simulink model "Simulink_Simulation"  (R2020a)
settings: Solver=ode23tb  StartTime=0.0  StopTime=10.0  RelTol=1e-3  EnableMultiTasking=on
undefined symbols (not defined in the file or in its folder): sigbuilder_block
libraries: powerlib x8
settings Model: Creator=LENOVO  LastModifiedBy=x64
settings DataIOCC: LimitDataPoints=on  SaveFormat=Array  ReturnWorkspaceOutputs=off
settings OptimizationCC: LifeSpan=inf
settings DebuggingCC: SolverPrmCheckMsg=warning  SFUnexpectedBacktrackingDiag=warning  SFNoUnconditionalDefaultTransitionDiag=warning  SFExecutionAtInitializationDiag=none  ArithmeticOperatorsInVariantConditions=warning
settings HardwareCC: ProdBitPerPointer=32  ProdBitPerSizeT=32  ProdBitPerPtrDiffT=32  ProdLargestAtomicFloat=None  ProdIntDivRoundTo=Undefined  ProdEndianess=Unspecified  ProdWordSize=32  ProdHWDeviceType=32-bit Generic
settings ModelReferenceCC: PropagateSignalLabelsOutOfModel=off
settings SFSimCC: SimUseLocalCustomCode=off  CustomCodeUndefinedFunction=UseInterfaceOnly
settings RTWCC: RTWUseLocalCustomCode=off
settings CodeAppCC: StateflowObjectComments=on
settings GRTTargetCC: TargetLangStandard=C89/C90 (ANSI)
settings ConfigComp: CovMetricSettings=dw  CovHtmlReporting=on  CovSaveCumulativeToWorkspaceVar=on  CovSaveSingleToWorkspaceVar=on  CovExternalEMLEnable=off  CovSFcnEnable=off
settings SimscapeCC: SimscapeNormalizeSystem=off

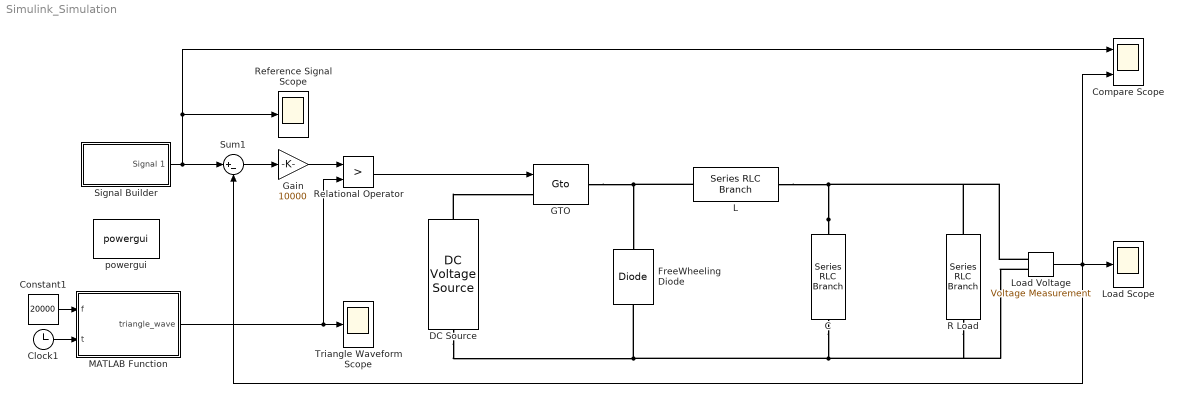
== system Simulink_Simulation ==
  "C " : powerlib/Elements/Series RLC Branch  LConnTagsString=__new0  RConnTagsString=__new0  BranchType=C  Resistance=1  Inductance=1e-3  SetiL0=off  InitialCurrent=0  Capacitance=(1e-6)*470  Setx0=off  InitialVoltage=0  Measurements=None
  Clock1 : Clock
  Compare Scope : Scope  NumInputPorts=2
  Constant1 : Constant  Value=20000
  "DC Source " : powerlib/Electrical Sources/DC Voltage Source  Amplitude=15  Measurements=None
  FreeWheeling Diode : powerlib/Power Electronics/Diode  Ron=0.01  Lon=1e-4  Vf=0.8  IC=0  UseSnubber=off  Rs=10000  Cs=1e-4  Measurements=off
  GTO : powerlib/Power Electronics/Gto  Ron=0.01  Lon=0.001  Vf=0.8  Tf=10e-6  Tt=20e-6  IC=0  Rs=10000  Cs=1e-5  Measurements=off
      settings: SourceProductBaseCode=PS
  Gain : Gain  Gain=10000
  L : powerlib/Elements/Series RLC Branch  LConnTagsString=__new0  RConnTagsString=__new0  BranchType=L  Resistance=1  Inductance=1e-4  SetiL0=off  InitialCurrent=0  Capacitance=1e-6  Setx0=off  InitialVoltage=0  Measurements=None
  Load Scope : Scope
  Load Voltage : powerlib/Measurements/Voltage Measurement  PhasorSimulation=off  OutputType=Complex  PSBequivalent=0
  "MATLAB Function " : MATLAB Function  TreatAsAtomicUnit=on
  R Load : powerlib/Elements/Series RLC Branch  LConnTagsString=__new0  RConnTagsString=__new0  BranchType=R  Resistance=25  Inductance=1e-3  SetiL0=off  InitialCurrent=0  Capacitance=1e-6  Setx0=off  InitialVoltage=0  Measurements=None
  Reference Signal Scope : Scope
  Relational Operator : RelationalOperator  Operator=>  OutDataTypeStr=boolean  RndMeth=Nearest
  "Signal Builder " : Subsystem  Tag=STV Subsys  LoadFcn=sigbuilder_block('load');  StartFcn=sigbuilder_block('start');  StopFcn=sigbuilder_block('stop');  ClipboardFcn=sigbuilder_block('clipboard');  mask(Sigbuilder block){tuvar=[0:10]}
      mask help: Simulink:masks:SigbuilderBlock_MD
      mask init:
      | if ~strcmp(get_param(bdroot(gcbh),'SimulationStatus'),'stopped') tuvar = sigbuilder_block('maskInit'); end
      settings: CopyFcn=sigbuilder_block('copy');  DeleteFcn=sigbuilder_block('delete');  ModelCloseFcn=sigbuilder_block('modelClose');  PreSaveFcn=sigbuilder_block('preSave');  PauseFcn=sigbuilder_block('pause');  ContinueFcn=sigbuilder_block('continue');  NameChangeFcn=sigbuilder_block('namechange');  OpenFcn=sigbuilder_block('open',[0 30 1152 561.6 ]);  CloseFcn=sigbuilder_block('close');
      mask Display: plot(0, 0, 100, 100,[2, 2, 32, 32, 2], [68, 8, 8, 68, 68],[32, 2], [38, 38], [32, 19, 2],[53, 60, 44], [32, 17, 17, 2],[16, 16, 31, 31]);txt = getActiveGroup(gcbh);text(2, 100, txt,'verticalAlignment', 'top');
  Sum1 : Sum  Inputs=|+-
  Triangle Waveform Scope : Scope
  powergui : powerlib/powergui  Priority=1  SimulationMode=Discrete  SampleTime=1e-006  frequency=60  Iterations=50  frequencyindice=0  Pbase=100e6  ErrMax=1e-4  UnitsV=kV  UnitsW=MW  buscounter=0  FunctionMessages=off  echomessages=off  EnableUseOfTLC=off  CurrentSourceSwitches=off  DisableSnubberDevices=off  DisableRonSwitches=off  DisableVfSwitches=off  DisplayEquations=off  AutomaticDiscreteSolvers=off  SolverType=Tustin  Interpol=off  ExternalGateDelay=off  methode=off  Ts=100  x0status=blocks  SPID=off  SwTol=0  HookPort=off  NonlinearTolerance=1e-4  nMaxIteration=100  ContinueOnMaxIteration=off  RestoreLinks=warning  ResistiveCurrentMeasurement=off  Frange=[0:2:500]  Ylog=off  Xlog=on  ShowGrid=off  save=off  variable=ZData  structure=0  ZoomFFT=off  StartTime=0.0  cycles=1  DisplayStyle=1  fundamental=60  FreqAxis=off  MaxFrequency=1000  frequencyindicesteady=1  RmsSteady=1  display=off
  wires:
  Clock1/1 -> "MATLAB Function "/2(t)
  Constant1/1 -> "MATLAB Function "/1(f)
  Load Voltage/1 -> Compare Scope/2, Load Scope/1, Sum1/2
  "Signal Builder "/1(Signal 1) -> Sum1/1, Reference Signal Scope/1, Compare Scope/1
  Sum1/1 -> Gain/1
  Relational Operator/1 -> GTO/1
  "MATLAB Function "/1(triangle_wave) -> Triangle Waveform Scope/1, Relational Operator/2
  Gain/1 -> Relational Operator/1
  connections:
  GTO/RConn1 -- L/LConn1 -- FreeWheeling Diode/RConn1
  "C "/LConn1 -- R Load/LConn1 -- Load Voltage/LConn1 -- L/RConn1
  "DC Source "/LConn1 -- R Load/RConn1 -- Load Voltage/LConn2 -- "C "/RConn1 -- FreeWheeling Diode/LConn1
  "DC Source "/RConn1 -- GTO/LConn1

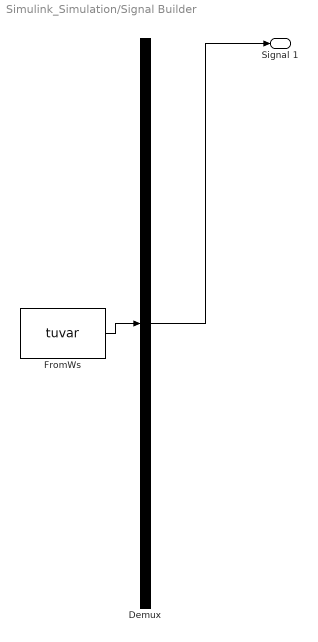
== system Simulink_Simulation/Signal Builder  ==
  Demux : Demux  Tag=STV Demux  Outputs=1
      settings: DisplayOption=none
  FromWs : FromWorkspace  Tag=STV FromWs  VariableName=tuvar
      SigBuilderData=|
      | common.afterFinalStr = 'Extrapolate'
      | common.sampleTime = 0
      | dataSet.timeRange = [0 10]
      | dataSet.name = 'Group 1'
      | sbobj.Groups.Name = 'Group 1'
      | sbobj.Groups.Signals.Name = 'Signal 1'
      | sbobj.Groups.Signals.XData = [0 3 3 4 6 6 8 8 10]
      | sbobj.Groups.Signals.YData = [12 12 6 6 6 4 4 8 8]
  Signal 1 : Outport  Tag=STV Outport
  wires:
  Demux/1 -> Signal 1/1
  FromWs/1 -> Demux/1

== matlab function Simulink_Simulation/MATLAB Function  ==
  data: f input; triangle_wave output; t input
function triangle_wave = Carrier_Generator(f, t)
%#codegen
% Generates a triangular carrier wave for PWM
% f: Switching Frequency (Hz)
% t: Simulation Clock Time (s)

amplitude = 1;
triangle_wave = 0;
multiplier = 1;

half_period = 1/(2*f);            % p
peak_time = half_period/2;        % tepe_zaman

cycle_time = mod(t, 2*half_period);   % t (Current position in full cycle)
local_time = mod(t, half_period);     % zaman (Current position in half cycle)

% Determine polarity based on cycle position
if (cycle_time < half_period)
    multiplier = -1;
else
    multiplier = 1;
end

% Generate Triangle Shape
if (local_time >= peak_time)
    % Falling edge calculation
    triangle_wave = multiplier * ((amplitude/peak_time) * (half_period - local_time));
else
    % Rising edge calculation
    triangle_wave = multiplier * ((amplitude/peak_time) * local_time);
end

return
